simulink model "iDesign_Converter_Dynamics"  (R2019a)
settings: Solver=FixedStepAuto  StartTime=0  StopTime=1000  FixedStep=9.5367e-06  RelTol=1e-3
libraries: simulink x4, Lib_Solve_SSNRSolverJC_TMATS x2
settings Model: Creator=pmatt  LastModifiedBy=pmatt
settings DataIOCC: SignalLoggingName=signalsOut

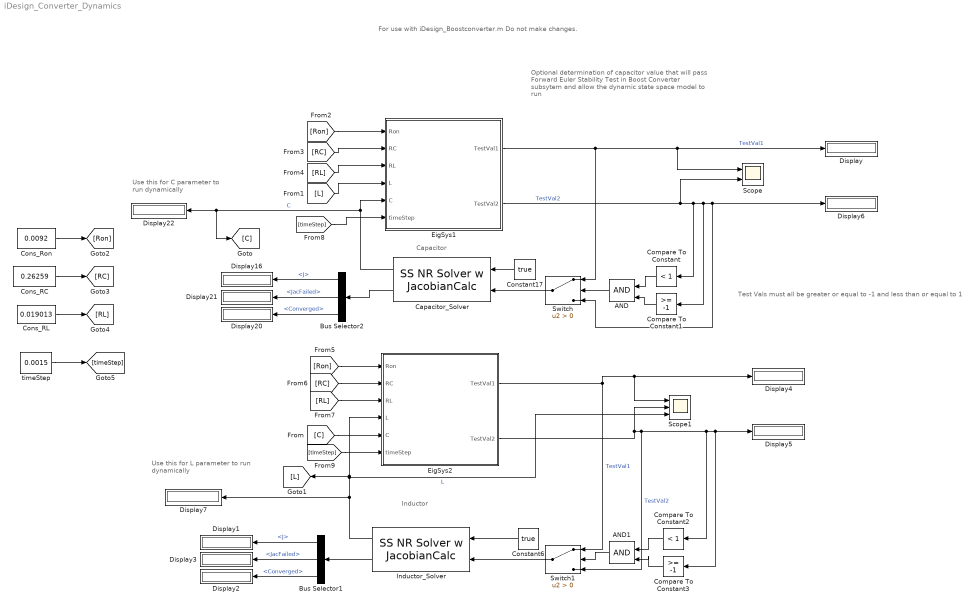
== system iDesign_Converter_Dynamics ==
  note: Capacitor
  note: Use this for C parameter to
      | run dynamically
  note: Optional determination of capacitor value
      | that will pass Forward Euler Stability Test
      | in Boost Converter subsytem and allow the dynamic
      | state space model to run
  note: Test Vals must all be greater or equal to -1 and less than or equal to 1
  note: For use with iDesign_Boostconverter.m
      | Do not make changes.
  note: Use this for L parameter to
      | run dynamically
  note: Inductor
  AND : Logic  IconShape=distinctive  AllPortsSameDT=off  OutDataTypeStr=boolean
  AND1 : Logic  IconShape=distinctive  AllPortsSameDT=off  OutDataTypeStr=boolean
  Bus Selector1 : BusSelector  OutputSignals=J,JacFailed,Converged
  Bus Selector2 : BusSelector  OutputSignals=J,JacFailed,Converged
  Capacitor_Solver : Lib_Solve_SSNRSolverJC_TMATS/SS NR Solver w JacobianCalc  SJac_Per_M=.005*[1; -1]  SNR_IC_M=5e-08  SNR_DX_M=1  SNR_Mx_M=1  SNR_Mn_M=1e-12  SJacobianAttempts_M=200  Cond_Limits_M=1
  Compare To Constant : simulink/Logic and Bit Operations/Compare To Constant  relop=<  const=1  OutDataTypeStr=boolean
  Compare To Constant1 : simulink/Logic and Bit Operations/Compare To Constant  relop=>=  const=-1  OutDataTypeStr=boolean
  Compare To Constant2 : simulink/Logic and Bit Operations/Compare To Constant  relop=<  const=1  OutDataTypeStr=boolean
  Compare To Constant3 : simulink/Logic and Bit Operations/Compare To Constant  relop=>=  const=-1  OutDataTypeStr=boolean
  Cons_RC : Constant  Value=0.26259
  Cons_RL : Constant  Value=0.019013
  Cons_Ron : Constant  Value=0.0092
  Constant17 : Constant  Value=true
  Constant6 : Constant  Value=true
  Display{,1..7,16,20..22} (12 alike) : Display
  EigSys1 : Subsystem
  EigSys2 : Subsystem
  Inductor_Solver : Lib_Solve_SSNRSolverJC_TMATS/SS NR Solver w JacobianCalc  SJac_Per_M=.005*[1; -1]  SNR_IC_M=5.9294e-05  SNR_DX_M=1  SNR_Mx_M=1  SNR_Mn_M=1e-12  SJacobianAttempts_M=200  Cond_Limits_M=.99999
  Scope : Scope  NumInputPorts=2
  Scope1 : Scope  NumInputPorts=3
  Switch : Switch  Criteria=u2 > Threshold
  Switch1 : Switch  Criteria=u2 > Threshold
  timeStep : Constant  Value=0.0015
  wires:
  Constant17/1 -> Capacitor_Solver/1
  Capacitor_Solver/2 -> Bus Selector2/1
  EigSys1/2(TestVal2) -> Scope/2, Compare To Constant1/1, Switch/3, Display6/1, Compare To Constant/1  "TestVal2"
  EigSys1/1(TestVal1) -> Scope/1, Display/1, Switch/1  "TestVal1"
  Bus Selector2/1 -> Display16/1  "<J>"
  Bus Selector2/2 -> Display21/1  "<JacFailed>"
  Bus Selector2/3 -> Display20/1  "<Converged>"
  AND/1 -> Switch/2
  Compare To Constant1/1 -> AND/2
  Compare To Constant/1 -> AND/1
  [L] -> EigSys1/4(L)
  Capacitor_Solver/1 -> EigSys1/5("C "), [C], Display22/1  "C"
  Switch/1 -> Capacitor_Solver/2
  [RC] -> EigSys2/2(RC)
  [RL] -> EigSys2/3(RL)
  [C] -> EigSys2/5("C ")
  Compare To Constant3/1 -> AND1/2
  AND1/1 -> Switch1/2
  Compare To Constant2/1 -> AND1/1
  Constant6/1 -> Inductor_Solver/1
  Bus Selector1/3 -> Display2/1  "<Converged>"
  Bus Selector1/2 -> Display3/1  "<JacFailed>"
  Bus Selector1/1 -> Display1/1  "<J>"
  Inductor_Solver/2 -> Bus Selector1/1
  Switch1/1 -> Inductor_Solver/2
  Inductor_Solver/1 -> [L], EigSys2/4(L), Scope1/3, Display7/1  "L"
  EigSys2/1(TestVal1) -> Display4/1, Scope1/1, Switch1/1  "TestVal1"
  EigSys2/2(TestVal2) -> Display5/1, Compare To Constant3/1, Compare To Constant2/1, Switch1/3, Scope1/2  "TestVal2"
  Cons_Ron/1 -> [Ron]
  Cons_RC/1 -> [RC]
  Cons_RL/1 -> [RL]
  [RL] -> EigSys1/3(RL)
  [RC] -> EigSys1/2(RC)
  [Ron] -> EigSys1/1(Ron)
  [Ron] -> EigSys2/1(Ron)
  timeStep/1 -> [timeStep]
  [timeStep] -> EigSys1/6(timeStep)
  [timeStep] -> EigSys2/6(timeStep)

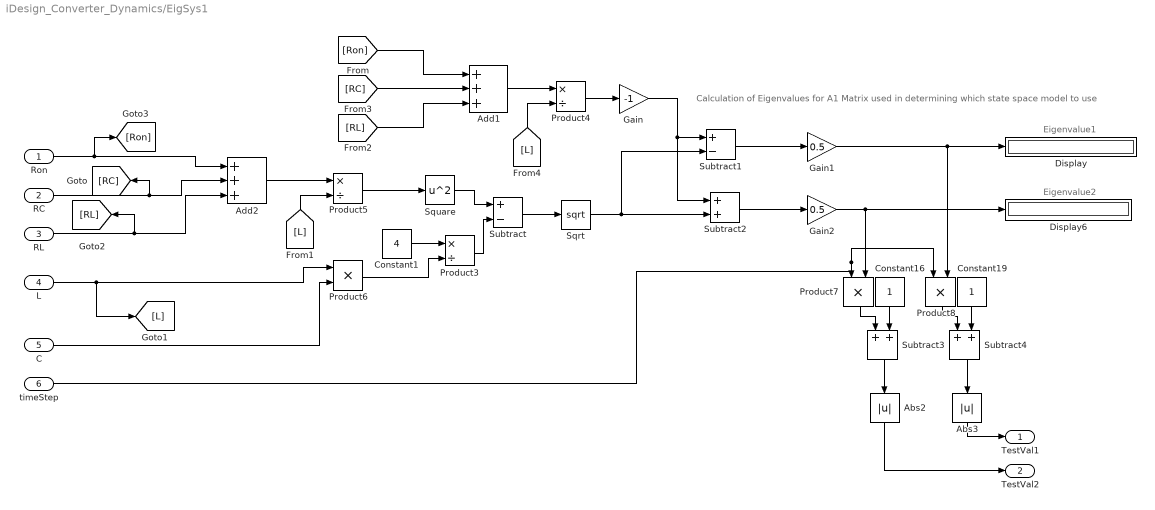
== system iDesign_Converter_Dynamics/EigSys1 ==
  note: Eigenvalue1
  note: Calculation of Eigenvalues for A1 Matrix used in determining which state space model to use
  note: Eigenvalue2
  Ron : Inport
  RC : Inport  Port=2
  RL : Inport  Port=3
  L : Inport  Port=4
  "C " : Inport  Port=5
  timeStep : Inport  Port=6
  Abs2 : Abs
  Abs3 : Abs
  Add1 : Sum  Inputs=+++
  Add2 : Sum  Inputs=+++
  Constant1 : Constant  Value=4
  Constant16 : Constant
  Constant19 : Constant
  Display : Display
  Display6 : Display
  Gain : Gain  Gain=-1
  Gain1 : Gain  Gain=0.5
  Gain2 : Gain  Gain=0.5
  Product3 : Product  Inputs=*/
  Product4 : Product  Inputs=*/
  Product5 : Product  Inputs=*/
  Product6 : Product
  Product7 : Product
  Product8 : Product
  Sqrt : Sqrt  OutputSignalType=complex  SaturateOnIntegerOverflow=on
  Square : Math  Operator=square  SaturateOnIntegerOverflow=on
  Subtract : Sum  Inputs=+-
  Subtract1 : Sum  Inputs=+-
  Subtract2 : Sum
  Subtract3 : Sum
  Subtract4 : Sum
  TestVal1 : Outport
  TestVal2 : Outport  Port=2
  wires:
  L/1 -> [L], Product6/1
  [RL] -> Add1/3
  Subtract4/1 -> Abs3/1
  Product4/1 -> Gain/1
  RC/1 -> Add2/2, [RC]
  Constant19/1 -> Subtract4/2
  Subtract3/1 -> Abs2/1
  timeStep/1 -> Product8/1, Product7/1
  Product8/1 -> Subtract4/1
  Product3/1 -> Subtract/2
  [Ron] -> Add1/1
  [L] -> Product4/2
  Constant1/1 -> Product3/1
  [L] -> Product5/2
  Gain2/1 -> Product7/2, Display6/1
  Gain1/1 -> Display/1, Product8/2
  RL/1 -> Add2/3, [RL]
  Abs2/1 -> TestVal2/1
  Constant16/1 -> Subtract3/2
  Product5/1 -> Square/1
  Product6/1 -> Product3/2
  Square/1 -> Subtract/1
  Subtract/1 -> Sqrt/1
  Sqrt/1 -> Subtract2/2, Subtract1/2
  Add2/1 -> Product5/1
  Add1/1 -> Product4/1
  Subtract2/1 -> Gain2/1
  Gain/1 -> Subtract1/1, Subtract2/1
  Subtract1/1 -> Gain1/1
  Ron/1 -> Add2/1, [Ron]
  Abs3/1 -> TestVal1/1
  Product7/1 -> Subtract3/1
  [RC] -> Add1/2
  "C "/1 -> Product6/2

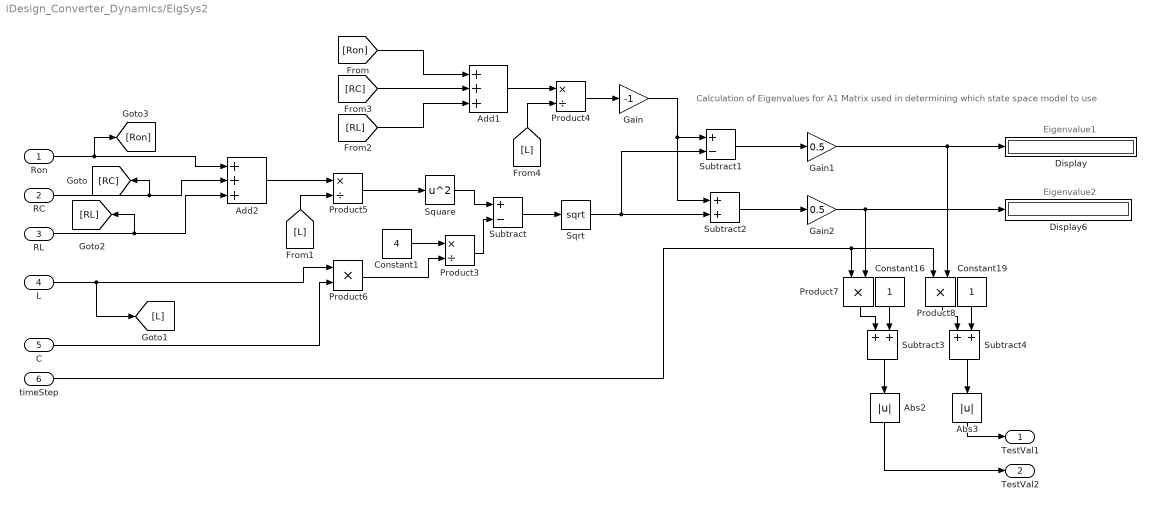
== system iDesign_Converter_Dynamics/EigSys2 ==
  note: Eigenvalue1
  note: Calculation of Eigenvalues for A1 Matrix used in determining which state space model to use
  note: Eigenvalue2
  Ron : Inport
  RC : Inport  Port=2
  RL : Inport  Port=3
  L : Inport  Port=4
  "C " : Inport  Port=5
  timeStep : Inport  Port=6
  Abs2 : Abs
  Abs3 : Abs
  Add1 : Sum  Inputs=+++
  Add2 : Sum  Inputs=+++
  Constant1 : Constant  Value=4
  Constant16 : Constant
  Constant19 : Constant
  Display : Display
  Display6 : Display
  Gain : Gain  Gain=-1
  Gain1 : Gain  Gain=0.5
  Gain2 : Gain  Gain=0.5
  Product3 : Product  Inputs=*/
  Product4 : Product  Inputs=*/
  Product5 : Product  Inputs=*/
  Product6 : Product
  Product7 : Product
  Product8 : Product
  Sqrt : Sqrt  OutputSignalType=complex  SaturateOnIntegerOverflow=on
  Square : Math  Operator=square  SaturateOnIntegerOverflow=on
  Subtract : Sum  Inputs=+-
  Subtract1 : Sum  Inputs=+-
  Subtract2 : Sum
  Subtract3 : Sum
  Subtract4 : Sum
  TestVal1 : Outport
  TestVal2 : Outport  Port=2
  wires:
  L/1 -> [L], Product6/1
  [RL] -> Add1/3
  Subtract4/1 -> Abs3/1
  Product4/1 -> Gain/1
  RC/1 -> Add2/2, [RC]
  Constant19/1 -> Subtract4/2
  Subtract3/1 -> Abs2/1
  timeStep/1 -> Product7/1, Product8/1
  Product8/1 -> Subtract4/1
  Product3/1 -> Subtract/2
  [Ron] -> Add1/1
  [L] -> Product4/2
  Constant1/1 -> Product3/1
  [L] -> Product5/2
  Gain2/1 -> Product7/2, Display6/1
  Gain1/1 -> Display/1, Product8/2
  RL/1 -> Add2/3, [RL]
  Abs2/1 -> TestVal2/1
  Constant16/1 -> Subtract3/2
  Product5/1 -> Square/1
  Product6/1 -> Product3/2
  Square/1 -> Subtract/1
  Subtract/1 -> Sqrt/1
  Sqrt/1 -> Subtract2/2, Subtract1/2
  Add2/1 -> Product5/1
  Add1/1 -> Product4/1
  Subtract2/1 -> Gain2/1
  Gain/1 -> Subtract1/1, Subtract2/1
  Subtract1/1 -> Gain1/1
  Ron/1 -> Add2/1, [Ron]
  Abs3/1 -> TestVal1/1
  Product7/1 -> Subtract3/1
  [RC] -> Add1/2
  "C "/1 -> Product6/2
